simulink model "dashboard"  (R2024b)
settings: Solver=VariableStepAuto  StartTime=0.0  StopTime=10.0  RelTol=1e-3
libraries: simulink x2
settings Model: Creator=balaj  LastModifiedBy=balaj

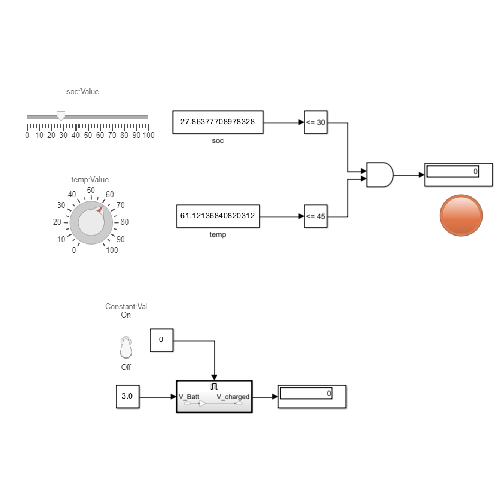
[thumbnail: Simulink's stored preview of the top-level diagram]
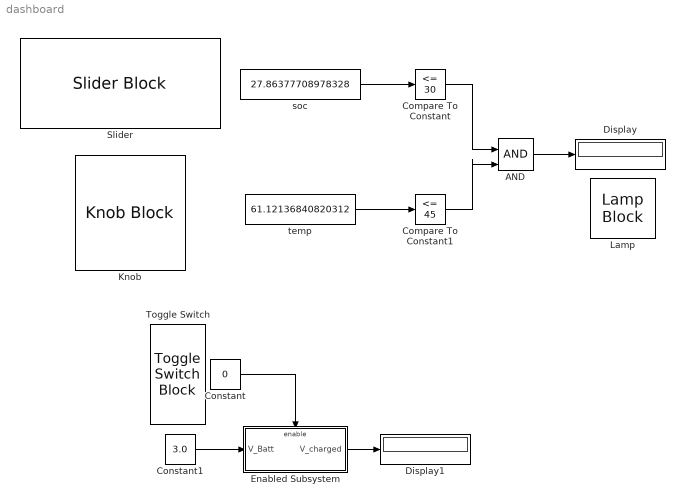
== system dashboard ==
  AND : Logic  IconShape=distinctive  AllPortsSameDT=off  OutDataTypeStr=boolean
  Compare To Constant : simulink/Logic and Bit Operations/Compare To Constant  relop=<=  const=30  OutDataTypeStr=boolean
  Compare To Constant1 : simulink/Logic and Bit Operations/Compare To Constant  relop=<=  const=45  OutDataTypeStr=boolean
  Constant : Constant  Value=0
  Constant1 : Constant  Value=3.0
  Display : Display
  Display1 : Display
  Enabled Subsystem : Subsystem  TreatAsAtomicUnit=on
  Knob : KnobBlock
  Lamp : LampBlock  LabelPosition=Hide
  Slider : SliderBlock
  Toggle Switch : ToggleSwitchBlock
      settings: Values={{'Off', 'On'}, [0 1]}
  soc : Constant  Value=27.86377708978328
  temp : Constant  Value=61.12136840820312
  wires:
  soc/1 -> Compare To Constant/1
  temp/1 -> Compare To Constant1/1
  Compare To Constant/1 -> AND/1
  Compare To Constant1/1 -> AND/2
  AND/1 -> Display/1
  Constant/1 -> Enabled Subsystem/Enable
  Constant1/1 -> Enabled Subsystem/1(V_Batt)
  Enabled Subsystem/1(V_charged) -> Display1/1

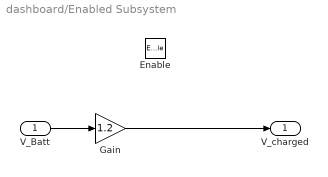
== system dashboard/Enabled Subsystem ==
  V_Batt : Inport
  Enable : EnablePort
  Gain : Gain  Gain=1.2
  V_charged : Outport
  wires:
  V_Batt/1 -> Gain/1
  Gain/1 -> V_charged/1
